simulink model "PhotodiodenMessschaltung"  (R2015b)
settings: Solver=VariableStepAuto  StartTime=0.0  StopTime=0.1  RelTol=1e-3
libraries: fl_lib x7, nesl_utility x2, elec_lib x1, dspxfrm3 x1
settings Model: Creator=lukaskiechle  LastModifiedBy=lukaskiechle

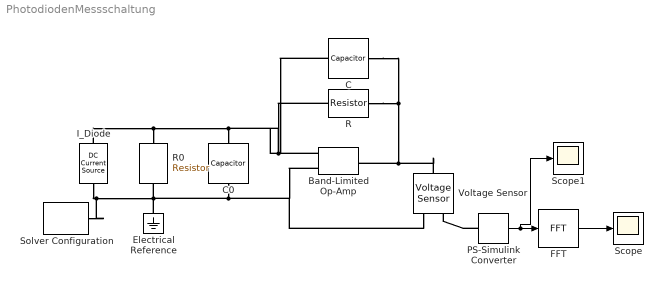
== system PhotodiodenMessschaltung ==
  Band-Limited Op-Amp : elec_lib/Integrated Circuits/Band-Limited Op-Amp  A=100000  Rin=1e6 Ohm  Rout=100 Ohm  Vmin=- 15 V  Vmax=15 V  Vdotmax=1000 V/s  f=1.6 Hz  V0=0 V
  C : fl_lib/Electrical/Electrical Elements/Capacitor  c=1 uF  r=1e-6 Ohm  g=0 1/Ohm  i_specify=off  i_priority=None  i=0 A  v_specify=off  v_priority=None  v=0 V  vc_specify=off  vc_priority=None  vc=0 V
  C0 : fl_lib/Electrical/Electrical Elements/Capacitor  c=10 pF  r=1e-6 Ohm  g=0 1/Ohm  i_specify=off  i_priority=None  i=0 A  v_specify=off  v_priority=None  v=0 V  vc_specify=off  vc_priority=None  vc=0 V
  Electrical Reference : fl_lib/Electrical/Electrical Elements/Electrical Reference
  FFT : dspxfrm3/FFT  FFTImplementation=Auto  CompMethod=Table lookup  TableOpt=NEW  TableOptActive=Speed  BitRevOrder=off  Normalize=off  InheritFFTLength=on  FFTLength=64  WrapInput=on  roundingMode=Floor  overflowMode=off  firstCoeffDataTypeStr=Inherit: Same word length as input  firstCoeffLastDataTypeStr=Inherit: Same word length as input  outputMin=[]  outputMax=[]
  I_Diode : fl_lib/Electrical/Electrical Sources/DC Current Source  i0=1 mA
  PS-Simulink Converter : nesl_utility/PS-Simulink Converter  PhysicalDomain=network_engine_domain  SubClassName=ps_output  LeftPortType=input  RightPortType=output  PseudoPeriodic=off  Frequencies=[]  Unit=1  AffineConversion=off
  R : fl_lib/Electrical/Electrical Elements/Resistor  R=100 MOhm  i_specify=off  i_priority=None  i=0 A  v_specify=off  v_priority=None  v=0 V
  R0 : fl_lib/Electrical/Electrical Elements/Resistor  R=1 GOhm  i_specify=off  i_priority=None  i=0 A  v_specify=off  v_priority=None  v=0 V
  Scope : Scope
  Scope1 : Scope
  Solver Configuration : nesl_utility/Solver Configuration  PhysicalDomain=network_engine_domain  SubClassName=solver  LeftPortType=input  RightPortType=generic  Accelerate=off  Tones=[]  Harmonics=[]  SimulateNoise=off  Profile=off  UseLocalSampling=off  EnableSwitchedLinearOptims=on  FrequencyDomain=off  UseCCode=off  RelTol=0.001  AbsTol=1e-06  MinStep=1e-09  ToWorkspace=off  RevertToSquareIcSolve=off  NumHomotopyIterations=100  PhasorMode=off  PhasorModeNumHarmonics=1  DoDC=on  ResidualTolerance=1e-09  UseLocalSolver=off  LocalSolverChoice=NE_BACKWARD_EULER_ADVANCER  LocalSolverSampleTime=0.001  DoFixedCost=off  MaxNonlinIter=3  MaxModeIter=2  LinearAlgebra=Sparse  DelaysMemoryBudget=1024  AutomaticFiltering=on  FilteringTimeConstant=0.001
  Voltage Sensor : fl_lib/Electrical/Electrical Sensors/Voltage Sensor
  wires:
  PS-Simulink Converter/1 -> Scope1/1, FFT/1
  FFT/1 -> Scope/1
  connections:
  I_Diode/RConn1 -- C/LConn1 -- R/LConn1 -- Band-Limited Op-Amp/LConn2 -- C0/RConn1 -- R0/RConn1
  I_Diode/LConn1 -- Solver Configuration/RConn1 -- Band-Limited Op-Amp/LConn1 -- Voltage Sensor/RConn2 -- C0/LConn1 -- R0/LConn1 -- Electrical Reference/LConn1
  R/RConn1 -- Band-Limited Op-Amp/RConn1 -- Voltage Sensor/LConn1 -- C/RConn1
  PS-Simulink Converter/LConn1 -- Voltage Sensor/RConn1
